simulink model "control_3dof"  (R2024b)
settings: configuration reference "prj_default_config" (kept outside this file)
values from neighbouring files (symbols this model uses):
  CONTROL_PARAM = Simulink.Parameter(CONTROL_PARAM_VALUE)    [control_init.m]
undefined symbols (not defined in the file or in its folder): CONTROL_CONST, DiscIntNeverNeededParam
libraries: mqlib x4, simulink x3
settings Model: Creator=yangyu  LastModifiedBy=yangyu
settings ConfigSetRef: SourceName=prj_default_config  SourceLocation=Base Workspace

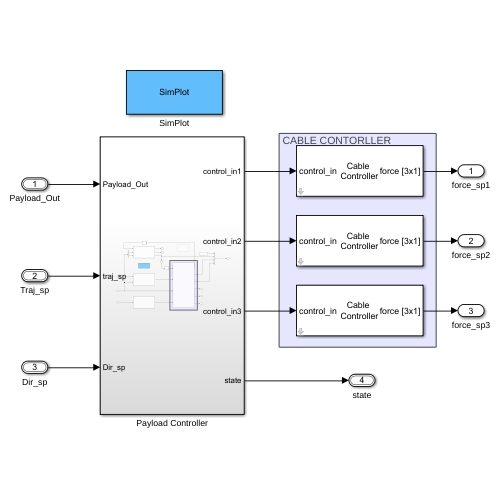
[thumbnail: Simulink's stored preview of the top-level diagram]
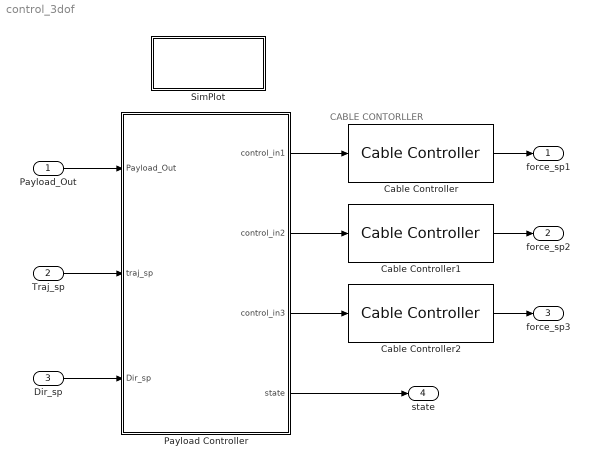
== system control_3dof ==
  note: CABLE CONTORLLER
  Payload_Out : Inport  OutDataTypeStr=Bus: Payload_Out_Bus
  Traj_sp : Inport  Port=2  OutDataTypeStr=Bus: TrajCmd_In_Bus
  Dir_sp : Inport  Port=3  OutDataTypeStr=Bus: DirCmd_In_Bus
  Cable Controller : mqlib/Cable Controller  Kq=CONTROL_PARAM.KQ  Kw=CONTROL_PARAM.KW  Ki=CONTROL_PARAM.KQI  mi=CONTROL_PARAM.MASS_UAV  li=CONTROL_PARAM.CABLE_LEN  beta_p=CONTROL_PARAM.ESO_PI  beta_v=CONTROL_PARAM.ESO_VI
  Cable Controller1 : mqlib/Cable Controller  Kq=CONTROL_PARAM.KQ  Kw=CONTROL_PARAM.KW  Ki=CONTROL_PARAM.KQI  mi=CONTROL_PARAM.MASS_UAV  li=CONTROL_PARAM.CABLE_LEN  beta_p=CONTROL_PARAM.ESO_PI  beta_v=CONTROL_PARAM.ESO_VI
  Cable Controller2 : mqlib/Cable Controller  Kq=CONTROL_PARAM.KQ  Kw=CONTROL_PARAM.KW  Ki=CONTROL_PARAM.KQI  mi=CONTROL_PARAM.MASS_UAV  li=CONTROL_PARAM.CABLE_LEN  beta_p=CONTROL_PARAM.ESO_PI  beta_v=CONTROL_PARAM.ESO_VI
  Payload Controller : Subsystem
  SimPlot : Subsystem
      settings: OpenFcn=run('simplot.m');
      mask Display: disp('SimPlot');
  force_sp1 : Outport  PortDimensions=3
  force_sp2 : Outport  Port=2  PortDimensions=3
  force_sp3 : Outport  Port=3  PortDimensions=3
  state : Outport  Port=4  OutDataTypeStr=Bus: Control_State_Bus
  wires:
  Traj_sp/1 -> Payload Controller/2(traj_sp)
  Cable Controller/1 -> force_sp1/1
  Cable Controller1/1 -> force_sp2/1
  Cable Controller2/1 -> force_sp3/1
  Payload Controller/1(control_in1) -> Cable Controller/1
  Payload Controller/2(control_in2) -> Cable Controller1/1
  Payload Controller/3(control_in3) -> Cable Controller2/1
  Payload_Out/1 -> Payload Controller/1(Payload_Out)
  Dir_sp/1 -> Payload Controller/3(Dir_sp)
  Payload Controller/4(state) -> state/1

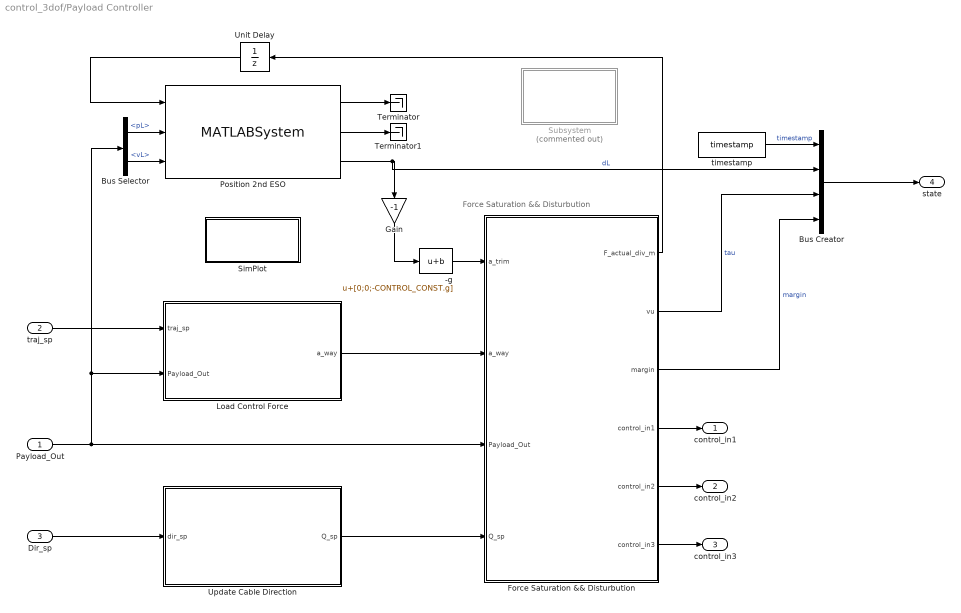
== system control_3dof/Payload Controller ==
  note: Force Saturation && Disturbution
  Payload_Out : Inport
  traj_sp : Inport  Port=2
  Dir_sp : Inport  Port=3
  -g : Bias  Bias=[0;0;-CONTROL_CONST.g]  SaturateOnIntegerOverflow=off
  Bus Creator : BusCreator  Inputs=4  OutDataTypeStr=Bus: Control_State_Bus
  Bus Selector : BusSelector  OutputSignals=pL,vL
  Force Saturation && Disturbution : MATLAB Function  TreatAsAtomicUnit=on  mask{mL=CONTROL_PARAM.MASS_LOAD, li=CONTROL_PARAM.CABLE_LEN, max_tension=CONTROL_PARAM.TENSION_MAX, min_tension=CONTROL_PARAM.TENSION_MIN}
  Gain : Gain  Gain=-1
  Load Control Force : Subsystem
  Position 2nd ESO : MATLABSystem  System=pos_2nd_eso  K_p=CONTROL_PARAM.ESO_PL  K_v=CONTROL_PARAM.ESO_VL  SampleTime=-1  SimulateUsing=Code generation
      mask Type: pos_2nd_eso
      mask Display:
      | disp('Position\n2nd Order ESO');
      | port_label('input',1,'acc');
      | port_label('input',2,'pos');
      | port_label('input',3,'vel');
      | port_label('output',1,'z1');
      | port_label('output',2,'z2');
      | port_label('output',3,'z3');
  SimPlot : Subsystem
      settings: OpenFcn=run('simplot.m');
      mask Display: disp('SimPlot');
  Subsystem : Subsystem  Commented=on
  Terminator : Terminator
  Terminator1 : Terminator
  Unit Delay : UnitDelay  SampleTime=-1  HasFrameUpgradeWarning=on
  Update Cable Direction : Subsystem
  timestamp : mqlib/timestamp  period=CONTROL_EXPORT.period
  control_in1 : Outport
  control_in2 : Outport  Port=2
  control_in3 : Outport  Port=3
  state : Outport  Port=4
  wires:
  Force Saturation && Disturbution/4(control_in1) -> control_in1/1
  Force Saturation && Disturbution/5(control_in2) -> control_in2/1
  Force Saturation && Disturbution/6(control_in3) -> control_in3/1
  Position 2nd ESO/3 -> Bus Creator/2, Gain/1  "dL"
  Bus Selector/2 -> Position 2nd ESO/3  "<vL>"
  Position 2nd ESO/1 -> Terminator/1
  Bus Selector/1 -> Position 2nd ESO/2  "<pL>"
  Position 2nd ESO/2 -> Terminator1/1
  -g/1 -> Force Saturation && Disturbution/1(a_trim)
  Dir_sp/1 -> Update Cable Direction/1(dir_sp)
  Update Cable Direction/1(Q_sp) -> Force Saturation && Disturbution/4(Q_sp)
  Gain/1 -> -g/1
  Bus Creator/1 -> state/1
  Load Control Force/1(a_way) -> Force Saturation && Disturbution/2(a_way)
  Force Saturation && Disturbution/1(F_actual_div_m) -> Unit Delay/1
  Unit Delay/1 -> Position 2nd ESO/1
  traj_sp/1 -> Load Control Force/1(traj_sp)
  Payload_Out/1 -> Load Control Force/2(Payload_Out), Bus Selector/1, Force Saturation && Disturbution/3(Payload_Out)
  Force Saturation && Disturbution/3(margin) -> Bus Creator/4  "margin"
  Force Saturation && Disturbution/2(vu) -> Bus Creator/3  "tau"
  timestamp/1 -> Bus Creator/1  "timestamp"

== system control_3dof/SimPlot ==

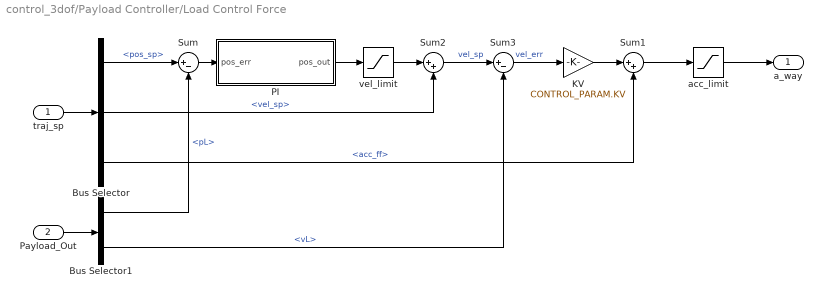
== system control_3dof/Payload Controller/Load Control Force ==
  traj_sp : Inport
  Payload_Out : Inport  Port=2
  Bus Selector : BusSelector  OutputSignals=pos_sp,vel_sp,acc_ff
  Bus Selector1 : BusSelector  OutputSignals=pL,vL
  KV : Gain  Gain=CONTROL_PARAM.KV
  PI : Subsystem
  Sum : Sum  Inputs=|+-
  Sum1 : Sum  Inputs=|++
  Sum2 : Sum  Inputs=|++
  Sum3 : Sum  Inputs=|+-
  acc_limit : Saturate  UpperLimit=3  LowerLimit=-3
  vel_limit : Saturate  UpperLimit=5  LowerLimit=-5
  a_way : Outport
  wires:
  Sum1/1 -> acc_limit/1
  traj_sp/1 -> Bus Selector/1
  Bus Selector/1 -> Sum/1  "<pos_sp>"
  Bus Selector1/1 -> Sum/2  "<pL>"
  Bus Selector/3 -> Sum1/2  "<acc_ff>"
  Payload_Out/1 -> Bus Selector1/1
  Bus Selector/2 -> Sum2/2  "<vel_sp>"
  Bus Selector1/2 -> Sum3/2  "<vL>"
  Sum3/1 -> KV/1  "vel_err"
  KV/1 -> Sum1/1
  Sum2/1 -> Sum3/1  "vel_sp"
  vel_limit/1 -> Sum2/1
  acc_limit/1 -> a_way/1
  Sum/1 -> PI/1(pos_err)
  PI/1(pos_out) -> vel_limit/1

== system control_3dof/Payload Controller/SimPlot ==

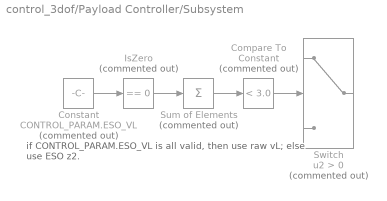
== system control_3dof/Payload Controller/Subsystem ==
  note: if CONTROL_PARAM.ESO_VL is all valid, then use raw vL;
      | else use ESO z2.
  Compare To Constant : simulink/Logic and Bit Operations/Compare To Constant  Commented=on  relop=<  const=3.0  OutDataTypeStr=boolean
  Constant : Constant  Commented=on  Value=CONTROL_PARAM.ESO_VL
  IsZero : simulink/Logic and Bit Operations/Compare To Zero  Commented=on  relop===  OutDataTypeStr=boolean
      settings: LibrarySourceBlock=|
      | simulink/Quick Insert/Logic and Bit
      | Operations/IsZero
  Sum of Elements : Sum  Commented=on  Inputs=+
  Switch : Switch  Commented=on  Criteria=u2 > Threshold  SaturateOnIntegerOverflow=off  InputSameDT=off
  wires:
  IsZero/1 -> Sum of Elements/1
  Sum of Elements/1 -> Compare To Constant/1
  Compare To Constant/1 -> Switch/2
  Constant/1 -> IsZero/1
  ? -> Switch/3

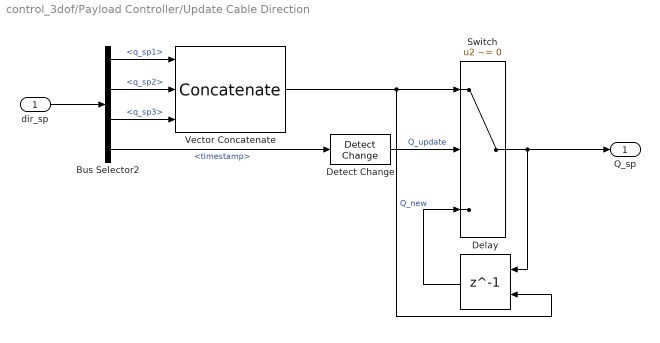
== system control_3dof/Payload Controller/Update Cable Direction ==
  dir_sp : Inport
  Bus Selector2 : BusSelector  OutputSignals=q_sp1,q_sp2,q_sp3,timestamp
  Delay : Delay  DelayLength=1  InitialConditionSource=Input port
      settings: InputPortMap=u0,p4
  Detect Change : simulink/Logic and Bit Operations/Detect Change  vinit=0  OutDataTypeStr=boolean
  Switch : Switch  Criteria=u2 ~= 0  SaturateOnIntegerOverflow=off  InputSameDT=off
  Vector Concatenate : Concatenate  NumInputs=3  Mode=Multidimensional array  ConcatenateDimension=2
  Q_sp : Outport
  wires:
  Detect Change/1 -> Switch/2  "Q_update"
  Vector Concatenate/1 -> Switch/1, Delay/2  "Q_new"
  Bus Selector2/4 -> Detect Change/1  "<timestamp>"
  Bus Selector2/2 -> Vector Concatenate/2  "<q_sp2>"
  dir_sp/1 -> Bus Selector2/1
  Bus Selector2/1 -> Vector Concatenate/1  "<q_sp1>"
  Bus Selector2/3 -> Vector Concatenate/3  "<q_sp3>"
  Switch/1 -> Delay/1, Q_sp/1
  Delay/1 -> Switch/3

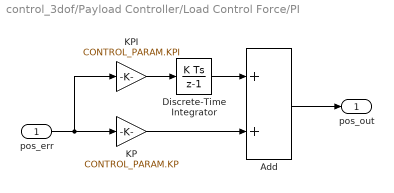
== system control_3dof/Payload Controller/Load Control Force/PI ==
  pos_err : Inport
  Add : Sum
  Discrete-Time Integrator : DiscreteIntegrator  gainval=1  SampleTime=-1  ICPrevOutput=DiscIntNeverNeededParam  ICPrevScaledInput=DiscIntNeverNeededParam
  KP : Gain  Gain=CONTROL_PARAM.KP
  KPI : Gain  Gain=CONTROL_PARAM.KPI
  pos_out : Outport
  wires:
  Discrete-Time Integrator/1 -> Add/1
  KPI/1 -> Discrete-Time Integrator/1
  pos_err/1 -> KPI/1, KP/1
  KP/1 -> Add/2
  Add/1 -> pos_out/1

== matlab function control_3dof/Payload Controller/Force Saturation && Disturbution ==
  data: F_actual_div_m output; vu output; margin output; a_trim input; a_way input; Payload_Out input Bus: Payload_Out_Bus; Q_sp input; control_in1 output Bus: Control_In_Bus; control_in2 output Bus: Control_In_Bus; control_in3 output Bus: Control_In_Bus; li parameter; max_tension parameter; min_tension parameter; mL parameter
function [F_actual_div_m, vu, margin, control_in1, control_in2, control_in3] = fcn(a_trim, a_way, Payload_Out, Q_sp, li, max_tension, min_tension, mL)
% id == 1
q_1 = Payload_Out.pL - Payload_Out.p_1;
q_1 = q_1 / norm(q_1);
w_1 = cross(q_1, (Payload_Out.vL - Payload_Out.v_1) / li);

% id == 2
q_2 = Payload_Out.pL - Payload_Out.p_2;
q_2 = q_2 / norm(q_2);
w_2 = cross(q_2, (Payload_Out.vL - Payload_Out.v_2) / li);

% id == 3
q_3 = Payload_Out.pL - Payload_Out.p_3;
q_3 = q_3 / norm(q_3);
w_3 = cross(q_3, (Payload_Out.vL - Payload_Out.v_3) / li);

Q = [q_1 q_2 q_3];
%% Force Saturation
% USE "PWAS"
F_trim = mL * a_trim;
F_way  = mL * a_way;
T_min = min_tension * ones(3, 1);
T_max = max_tension * ones(3, 1);
[vu, F_actual] = PWAS(F_trim, F_way, Q, T_min, T_max);

% adjust aL
aL_sp = [0;0;-9.8] + (F_actual - F_trim) / mL;

F_actual_div_m = F_actual / mL;
%% Margin Calculation
margin = margin_lp(F_trim, -Q, T_min, T_max);

%% Force Disturbution
control_in1.timestamp = uint64(1);
control_in1.vforce = vu(1) * q_1;
control_in1.q_sp = Q_sp(:, 1);
control_in1.q = q_1;
control_in1.w = w_1;
control_in1.ai_sp = aL_sp;
control_in1.pi = Payload_Out.p_1;
control_in1.vi = Payload_Out.v_1;

control_in2.timestamp = uint64(1);
control_in2.vforce = vu(2) * q_2;
control_in2.q_sp = Q_sp(:, 2);
control_in2.q = q_2;
control_in2.w = w_2;
control_in2.ai_sp = aL_sp;
control_in2.pi = Payload_Out.p_2;
control_in2.vi = Payload_Out.v_2;

control_in3.timestamp = uint64(1);
control_in3.vforce = vu(3) * q_3;
control_in3.q_sp = Q_sp(:, 3);
control_in3.q = q_3;
control_in3.w = w_3;
control_in3.ai_sp = aL_sp;
control_in3.pi = Payload_Out.p_3;
control_in3.vi = Payload_Out.v_3;
end
